simulink model "PCCI"  (R2024b)
settings: Solver=FixedStepDiscrete  StartTime=0.0  StopTime=10.0  FixedStep=0.001  RelTol=1e-3
settings Model: Creator=LENOVO  LastModifiedBy=LENOVO
settings OptimizationCC: DefaultParameterBehavior=Inlined  EnhancedBackFolding=on  PassReuseOutputArgsAs=Individual arguments  ZeroExternalMemoryAtStartup=off  ZeroInternalMemoryAtStartup=off  OptimizeBlockOrder=speed  DifferentSizesBufferReuse=on  OptimizationCustomize=off  EfficientTunableParamExpr=on
settings DebuggingCC: ParameterTunabilityLossMsg=error
settings SFSimCC: MATLABDynamicMemAlloc=off
settings RTWCC: Description=Embedded Coder  SystemTargetFile=ert.tlc  GenCodeOnly=on  TemplateMakefile=ert_default_tmf  GenerateReport=on  LaunchReport=on  GenerateCodeMetricsReport=on  GPUComputeCapability=3.5
settings CodeAppCC: ForceParamTrailComments=on  IgnoreCustomStorageClasses=off  OperatorAnnotations=on  SimulinkDataObjDesc=on  SFDataObjDesc=on  InsertBlockDesc=on
settings ERTTargetCC: TargetLangStandard=C99 (ISO)  GenerateSampleERTMain=on  ERTCustomFileTemplate=example_file_process.tlc

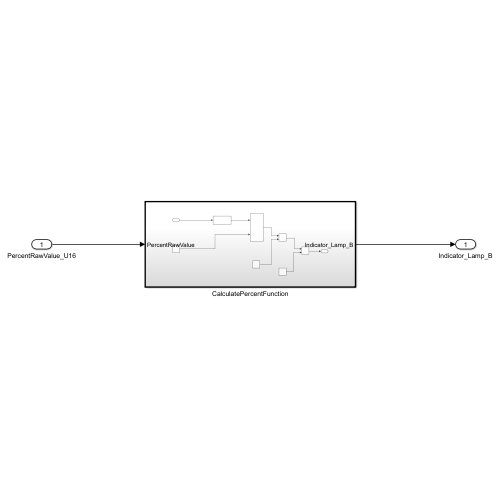
[thumbnail: Simulink's stored preview of the top-level diagram]
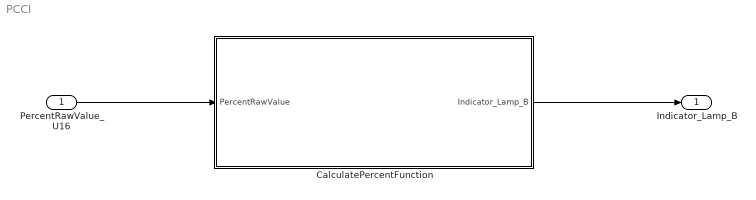
== system PCCI ==
  PercentRawValue_U16 : Inport
  CalculatePercentFunction : Subsystem  TreatAsAtomicUnit=on
      settings: RTWFcnNameOpts=Use subsystem name  RTWFileNameOpts=Use subsystem name
  Indicator_Lamp_B : Outport  OutDataTypeStr=boolean
  wires:
  PercentRawValue_U16/1 -> CalculatePercentFunction/1(PercentRawValue)
  CalculatePercentFunction/1(Indicator_Lamp_B) -> Indicator_Lamp_B/1

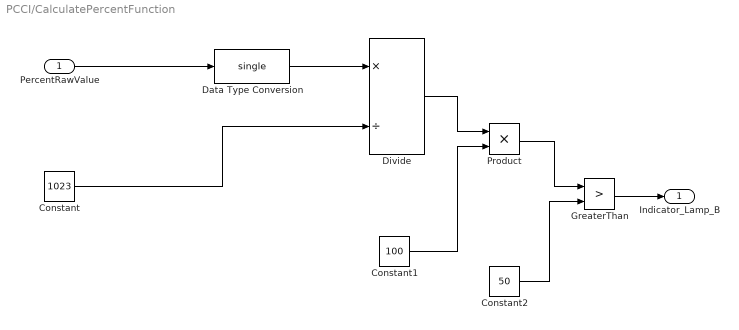
== system PCCI/CalculatePercentFunction ==
  PercentRawValue : Inport
  Constant : Constant  Value=1023  OutDataTypeStr=single
  Constant1 : Constant  Value=100  OutDataTypeStr=uint8
  Constant2 : Constant  Value=50  OutDataTypeStr=uint8
  Data Type Conversion : DataTypeConversion  OutDataTypeStr=single  SaturateOnIntegerOverflow=off  RndMeth=Floor
  Divide : Product  Inputs=*/
  GreaterThan : RelationalOperator  Operator=>  OutDataTypeStr=boolean  RndMeth=Simplest  InputSameDT=off
  Product : Product
  Indicator_Lamp_B : Outport  OutDataTypeStr=boolean
  wires:
  PercentRawValue/1 -> Data Type Conversion/1
  Constant/1 -> Divide/2
  Data Type Conversion/1 -> Divide/1
  Divide/1 -> Product/1
  Constant1/1 -> Product/2
  Product/1 -> GreaterThan/1
  Constant2/1 -> GreaterThan/2
  GreaterThan/1 -> Indicator_Lamp_B/1
